simulink model "sampleModel1921"  (R2023a)
settings: Solver=VariableStepAuto  StartTime=0.0  StopTime=10.0  RelTol=1e-3
libraries: hdlsllib x3, simulink x2
settings Model: Creator=user1  LastModifiedBy=user1

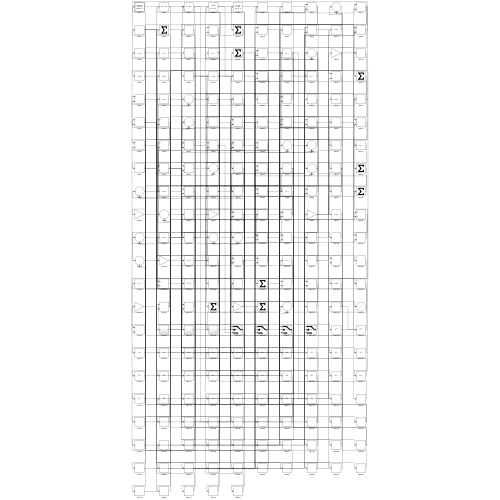
[thumbnail: Simulink's stored preview of the top-level diagram]
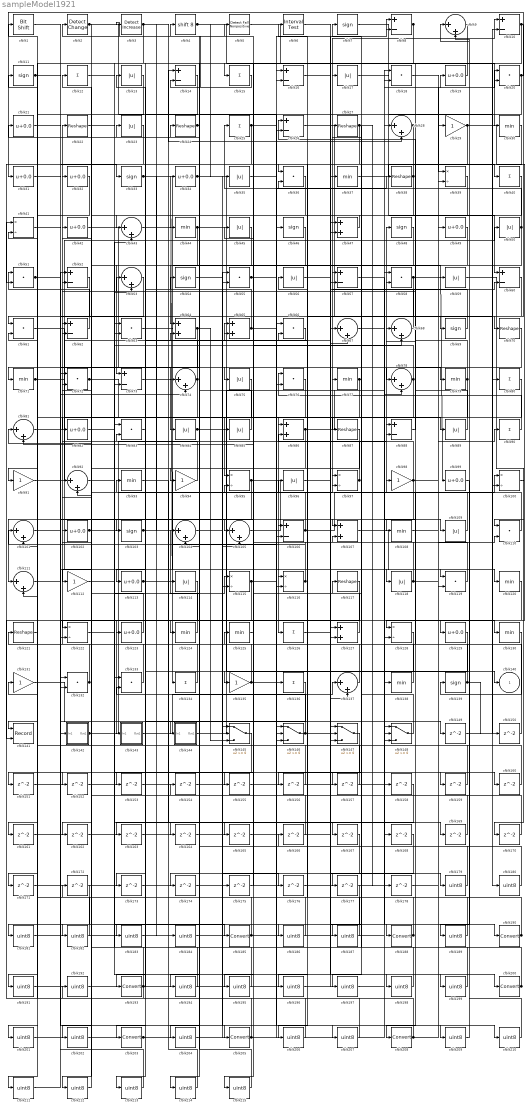
== system sampleModel1921 ==
  cfblk1 : hdlsllib/Logic and Bit Operations/Bit Shift  mode=Shift Left Logical  N=0
  cfblk{8,10,14,16,26,52,57,60,62,73,88,106} (12 alike) : Sum  Inputs=+-
  cfblk{39,41,95,97,100,115..116,122,128} (9 alike) : Product  Inputs=*/  RndMeth=Zero  SaturateOnIntegerOverflow=on
  cfblk{9,28,43,53,67..68,74,78,81,92,101,104..105,111,137} (15 alike) : Sum  Inputs=|++
  cfblk{19,21,31..32,34,42,49,82,99,102,113,123,129} (13 alike) : Bias  Bias=0.0  SaturateOnIntegerOverflow=off
  cfblk{7,11,33,46,48,54,69,103,139} (9 alike) : Signum
  cfblk{47,64..65,86,107,127} (6 alike) : Sum
  cfblk{30,37,44,71,77,79,93,108,120,124..125,130,138} (13 alike) : MinMax
  cfblk{13,17,23,35,45,50,56,59,75,84..85,89,96,109,114,118} (16 alike) : Abs  SaturateOnIntegerOverflow=off
  cfblk{18,20,36,51,55,58,61,63,66,72,76,83,110,119,132..133} (16 alike) : DotProduct  OutDataTypeStr=Inherit: Inherit via internal rule
  cfblk{29,91,94,98,112,131,135} (7 alike) : Gain
  cfblk{22,24,27,38,70,87,117,121} (8 alike) : Reshape
  cfblk{12,15,25,40,80,90,126,134,136} (9 alike) : Sum  Inputs=+
  cfblk141 : Record  FileSettingsInternal="{\"entries\":[{\"content\":{\"excelSettings\":{\"content\":{},\"type\":\"Streamout.ExcelSettings\"}},\"type\":\"Streamout.FileSettingStorage\",\"uuid\":\"\"}],\"packageUris\":[\"http:\\/\\/schema.mathworks.com\\/mf0\\/streamout_blocks\\/R2020a\"],\"version\":\"1.0\"}"  Layout=[1 1]  SignalsInternal="{\"entries\":[{\"content\":{\"signals\":[{\"content\":{\"blockPath\":[],\"dimensions\":[1],\"domain\":\"\",\"lineColor\":\"#a2142f\",\"plots\":[1],\"port\":1,\"signalID\":5141,\"signalName\":\"XY Graph:1\"},\"type\":\"RecordBlkView.Signal\",\"uuid\":\"\"},{\"content\":{\"blockPath\":[],\"dimensions\":[1],\"domain\":\"\",\"lineColor\":\"#139fff\",\"plots\":[1],\"port\":2,\"signalID\":5144,\"signalName\":\"XY Graph:2\"},\"type\":\"RecordBlkView.Signal\",\"uuid\":\"\"}]},\"type\":\"RecordBlkView.InputSignals\",\"uuid\":\"\"}],\"packageUris\":[\"http:\\/\\/schema.mathworks.com\\/mf0\\/streamout_blocks\\/R2020a\"],\"version\":\"1.0\"}"  VisualizationBindings="{\"xyplotplugin\":{\"info\":[{\"series\":[{\"bindingParametersList\":[{\"parameter\":\"X-Axis\",\"signalID\":5141,\"signalName\":\"XY Graph:1\"},{\"parameter\":\"Y-Axis\",\"signalID\":5144,\"signalName\":\"XY Graph:2\"}],\"seriesID\":61603}],\"subplotID\":1}]}}"  CompatibilityTag=XY  st=-1
  cfblk142 : Subsystem
      settings: LibrarySourceBlock=|
      | hdlsllib/Ports &
      | Subsystems/Subsystem
  cfblk143 : Subsystem
      settings: LibrarySourceBlock=|
      | hdlsllib/Ports &
      | Subsystems/Subsystem
  cfblk144 : Subsystem
      settings: LibrarySourceBlock=|
      | hdlsllib/Ports &
      | Subsystems/Subsystem
  cfblk{145..148} (4 alike) : Switch  SaturateOnIntegerOverflow=off  InputSameDT=off
  cfblk{149..178} (30 alike) : Delay  SampleTime=1
  cfblk{179..184,186..187,189,191..192,194..199,201..202,204,206..207,209..215} (29 alike) : DataTypeConversion  OutDataTypeStr=uint8  SaturateOnIntegerOverflow=off  RndMeth=Floor
  cfblk{185,188,190,193,200,203,205,208} (8 alike) : DataTypeConversion  SaturateOnIntegerOverflow=off  RndMeth=Floor
  cfblk2 : simulink/Logic and Bit Operations/Detect Change  vinit=0  OutDataTypeStr=boolean
      settings: LibrarySourceBlock=|
      | hdlsllib/Logic and Bit
      | Operations/Detect
      | Change
  cfblk3 : simulink/Logic and Bit Operations/Detect Increase  vinit=0.0  OutDataTypeStr=boolean
      settings: LibrarySourceBlock=|
      | hdlsllib/Logic and Bit
      | Operations/Detect
      | Increase
  cfblk4 : ArithShift  BitShiftNumber=8
  cfblk5 : hdlsllib/Logic and Bit Operations/Detect Fall Nonpositive  vinit=0  OutDataTypeStr=boolean
  cfblk6 : hdlsllib/Logic and Bit Operations/Interval Test  IntervalClosedRight=on  uplimit=0.5  IntervalClosedLeft=on  lowlimit=-0.5  OutDataTypeStr=boolean
  cfblk140 : Outport  VectorParamsAs1DForOutWhenUnconnected=off
  wires:
  cfblk65/1 -> cfblk23/1, cfblk38/1
  cfblk106/1 -> cfblk100/1, cfblk81/1
  cfblk142/1(Out1) -> cfblk10/1, cfblk115/1
  cfblk33/1 -> cfblk134/1, cfblk59/1
  cfblk103/1 -> cfblk97/1, cfblk34/1
  cfblk79/1 -> cfblk26/1, cfblk145/2, cfblk212/1
  cfblk2/1 -> cfblk46/1, cfblk202/1
  cfblk102/1 -> cfblk48/1, cfblk68/2, cfblk169/1
  cfblk132/1 -> cfblk22/1, cfblk101/2
  cfblk50/1 -> cfblk25/1, cfblk115/2
  cfblk20/1 -> cfblk31/1, cfblk44/1
  cfblk133/1 -> cfblk32/1
  cfblk63/1 -> cfblk120/1
  cfblk7/1 -> cfblk60/1
  cfblk42/1 -> cfblk78/1
  cfblk16/1 -> cfblk200/1
  cfblk19/1 -> cfblk15/1
  cfblk109/1 -> cfblk42/1
  cfblk85/1 -> cfblk21/1
  cfblk59/1 -> cfblk110/1
  cfblk95/1 -> cfblk111/1, cfblk127/1
  cfblk53/1 -> cfblk61/1
  cfblk15/1 -> cfblk3/1
  cfblk78/1 -> cfblk126/1, cfblk5/1
  cfblk74/1 -> cfblk13/1, cfblk122/2
  cfblk34/1 -> cfblk140/1, cfblk176/1
  cfblk27/1 -> cfblk177/1, cfblk178/1, cfblk195/1
  cfblk47/1 -> cfblk43/1
  cfblk1/1 -> cfblk142/1(In1)
  cfblk124/1 -> cfblk104/1
  cfblk38/1 -> cfblk36/1, cfblk57/2
  cfblk61/1 -> cfblk116/1
  cfblk43/1 -> cfblk75/1
  cfblk91/1 -> cfblk50/1
  cfblk41/1 -> cfblk205/1
  cfblk119/1 -> cfblk2/1
  cfblk134/1 -> cfblk62/1
  cfblk49/1 -> cfblk64/1
  cfblk117/1 -> cfblk143/1(In1)
  cfblk24/1 -> cfblk4/1, cfblk164/1
  cfblk144/1(Out1) -> cfblk28/1
  cfblk29/1 -> cfblk128/1, cfblk51/2, cfblk174/1
  cfblk114/1 -> cfblk124/1
  cfblk58/1 -> cfblk99/1, cfblk186/1
  cfblk97/1 -> cfblk77/1, cfblk86/2
  cfblk94/1 -> cfblk62/2
  cfblk143/1(Out1) -> cfblk137/1
  cfblk8/1 -> cfblk94/1, cfblk63/2
  cfblk113/1 -> cfblk26/2, cfblk88/2
  cfblk116/1 -> cfblk101/1, cfblk81/2
  cfblk131/1 -> cfblk144/1(In1)
  cfblk28/1 -> cfblk112/1, cfblk74/1
  cfblk39/1 -> cfblk105/1
  cfblk72/1 -> cfblk95/1, cfblk106/2, cfblk87/1
  cfblk44/1 -> cfblk147/2, cfblk122/1
  cfblk4/1 -> cfblk30/1, cfblk35/1
  cfblk55/1 -> cfblk109/1, cfblk128/2
  cfblk22/1 -> cfblk130/1
  cfblk21/1 -> cfblk33/1
  cfblk31/1 -> cfblk69/1
  cfblk123/1 -> cfblk102/1
  cfblk69/1 -> cfblk17/1
  cfblk88/1 -> cfblk68/1
  cfblk96/1 -> cfblk60/2
  cfblk120/1 -> cfblk129/1
  cfblk71/1 -> cfblk58/2, cfblk43/2
  cfblk127/1 -> cfblk65/1
  cfblk84/1 -> cfblk20/1, cfblk54/1
  cfblk66/1 -> cfblk64/2
  cfblk62/1 -> cfblk11/1
  cfblk37/1 -> cfblk40/1
  cfblk45/1 -> cfblk73/1
  cfblk86/1 -> cfblk19/1, cfblk162/1, cfblk163/1
  cfblk13/1 -> cfblk141/1
  cfblk105/1 -> cfblk107/1
  cfblk146/1 -> cfblk66/2, cfblk133/2, cfblk8/2
  cfblk52/1 -> cfblk71/1
  cfblk137/1 -> cfblk53/1
  cfblk135/1 -> cfblk146/3, cfblk51/1
  cfblk56/1 -> cfblk188/1
  cfblk67/1 -> cfblk190/1
  cfblk77/1 -> cfblk85/1, cfblk187/1
  cfblk139/1 -> cfblk98/1, cfblk150/1
  cfblk17/1 -> cfblk80/1
  cfblk18/1 -> cfblk39/1
  cfblk107/1 -> cfblk119/1
  cfblk83/1 -> cfblk193/1
  cfblk101/1 -> cfblk118/1
  cfblk136/1 -> cfblk203/1
  cfblk115/1 -> cfblk8/1, cfblk141/2, cfblk204/1
  cfblk26/1 -> cfblk100/2
  cfblk108/1 -> cfblk49/1
  cfblk40/1 -> cfblk103/1
  cfblk81/1 -> cfblk86/1
  cfblk25/1 -> cfblk89/1, cfblk82/1
  cfblk57/1 -> cfblk138/1
  cfblk10/1 -> cfblk135/1, cfblk70/1, cfblk113/1
  cfblk64/1 -> cfblk91/1, cfblk145/3
  cfblk90/1 -> cfblk76/1
  cfblk82/1 -> cfblk73/2
  cfblk70/1 -> cfblk108/1
  cfblk11/1 -> cfblk123/1, cfblk79/1, cfblk210/1
  cfblk118/1 -> cfblk110/2, cfblk96/1
  cfblk130/1 -> cfblk139/1
  cfblk68/1 -> cfblk7/1
  cfblk92/1 -> cfblk185/1
  cfblk9/1 -> cfblk208/1
  cfblk3/1 -> cfblk28/2, cfblk161/1, cfblk184/1
  cfblk110/1 -> cfblk88/1
  cfblk125/1 -> cfblk45/1
  cfblk126/1 -> cfblk47/1
  cfblk89/1 -> cfblk52/2
  cfblk73/1 -> cfblk84/1
  cfblk51/1 -> cfblk106/1, cfblk74/2
  cfblk148/1 -> cfblk57/1
  cfblk138/1 -> cfblk125/1
  cfblk98/1 -> cfblk90/1, cfblk36/2, cfblk148/2, cfblk20/2
  cfblk111/1 -> cfblk149/1
  cfblk149/1 -> cfblk10/2
  cfblk150/1 -> cfblk1/1
  cfblk76/1 -> cfblk151/1
  cfblk151/1 -> cfblk66/1
  cfblk36/1 -> cfblk152/1
  cfblk152/1 -> cfblk58/1
  cfblk80/1 -> cfblk153/1
  cfblk153/1 -> cfblk146/2
  cfblk154/1 -> cfblk78/2
  cfblk46/1 -> cfblk155/1
  cfblk155/1 -> cfblk147/1
  cfblk30/1 -> cfblk156/1
  cfblk156/1 -> cfblk52/1
  cfblk60/1 -> cfblk157/1
  cfblk157/1 -> cfblk61/2
  cfblk112/1 -> cfblk159/1
  cfblk159/1 -> cfblk107/2
  cfblk122/1 -> cfblk160/1
  cfblk160/1 -> cfblk146/1
  cfblk161/1 -> cfblk47/2
  cfblk162/1 -> cfblk53/2
  cfblk163/1 -> cfblk116/2
  cfblk164/1 -> cfblk147/3
  cfblk129/1 -> cfblk165/1
  cfblk166/1 -> cfblk72/2
  cfblk93/1 -> cfblk167/1
  cfblk169/1 -> cfblk95/2
  cfblk100/1 -> cfblk170/1
  cfblk170/1 -> cfblk97/2
  cfblk145/1 -> cfblk171/1
  cfblk171/1 -> cfblk105/2
  cfblk128/1 -> cfblk173/1
  cfblk173/1 -> cfblk39/2
  cfblk174/1 -> cfblk127/2
  cfblk104/1 -> cfblk175/1
  cfblk175/1 -> cfblk65/2
  cfblk176/1 -> cfblk18/2
  cfblk178/1 -> cfblk119/2
  cfblk6/1 -> cfblk179/1
  cfblk179/1 -> cfblk114/1
  cfblk5/1 -> cfblk180/1
  cfblk180/1 -> cfblk6/1
  cfblk121/1 -> cfblk181/1
  cfblk181/1 -> cfblk55/1
  cfblk23/1 -> cfblk182/1
  cfblk182/1 -> cfblk121/1
  cfblk158/1 -> cfblk183/1
  cfblk183/1 -> cfblk55/2
  cfblk184/1 -> cfblk158/1
  cfblk185/1 -> cfblk104/2, cfblk137/2
  cfblk186/1 -> cfblk92/1
  cfblk187/1 -> cfblk92/2
  cfblk188/1 -> cfblk72/1, cfblk111/2
  cfblk99/1 -> cfblk189/1
  cfblk189/1 -> cfblk56/1
  cfblk190/1 -> cfblk166/1, cfblk63/1
  cfblk32/1 -> cfblk191/1
  cfblk191/1 -> cfblk67/1
  cfblk192/1 -> cfblk67/2
  cfblk193/1 -> cfblk192/1, cfblk37/1, cfblk133/1, cfblk93/1
  cfblk167/1 -> cfblk194/1
  cfblk194/1 -> cfblk83/1
  cfblk195/1 -> cfblk83/2
  cfblk168/1 -> cfblk196/1
  cfblk196/1 -> cfblk148/1
  cfblk48/1 -> cfblk197/1
  cfblk197/1 -> cfblk168/1
  cfblk12/1 -> cfblk198/1
  cfblk198/1 -> cfblk117/1
  cfblk35/1 -> cfblk199/1
  cfblk199/1 -> cfblk12/1
  cfblk200/1 -> cfblk27/1, cfblk24/1
  cfblk177/1 -> cfblk201/1
  cfblk201/1 -> cfblk16/1
  cfblk202/1 -> cfblk16/2
  cfblk203/1 -> cfblk148/3, cfblk76/2, cfblk145/1
  cfblk204/1 -> cfblk136/1
  cfblk205/1 -> cfblk154/1, cfblk18/1
  cfblk147/1 -> cfblk206/1
  cfblk206/1 -> cfblk41/1
  cfblk165/1 -> cfblk207/1
  cfblk207/1 -> cfblk41/2
  cfblk208/1 -> cfblk29/1, cfblk131/1
  cfblk54/1 -> cfblk209/1
  cfblk209/1 -> cfblk9/1
  cfblk210/1 -> cfblk9/2
  cfblk172/1 -> cfblk211/1
  cfblk211/1 -> cfblk132/2
  cfblk212/1 -> cfblk172/1
  cfblk14/1 -> cfblk213/1
  cfblk213/1 -> cfblk132/1
  cfblk75/1 -> cfblk214/1
  cfblk214/1 -> cfblk14/1
  cfblk87/1 -> cfblk215/1
  cfblk215/1 -> cfblk14/2

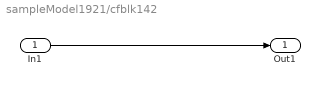
== system sampleModel1921/cfblk142 ==
  In1 : Inport
  Out1 : Outport
  wires:
  In1/1 -> Out1/1

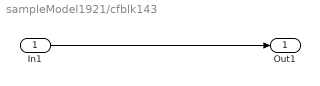
== system sampleModel1921/cfblk143 ==
  In1 : Inport
  Out1 : Outport
  wires:
  In1/1 -> Out1/1

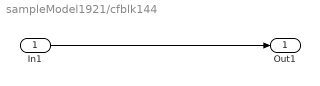
== system sampleModel1921/cfblk144 ==
  In1 : Inport
  Out1 : Outport
  wires:
  In1/1 -> Out1/1
